simulink model "Stop_Model"  (R2023a)
settings: Solver=VariableStepAuto  StartTime=0.0  StopTime=10.0  RelTol=1e-3
libraries: TimeSharedLib x2, NSA_DEVS_SINKS_ATOMIC x2, NSA_DEVS_SOURCES_ATOMIC x1, NSA_DEVS_LOGISTICS_ATOMIC x1
settings Model: Creator=david  LastModifiedBy=peter

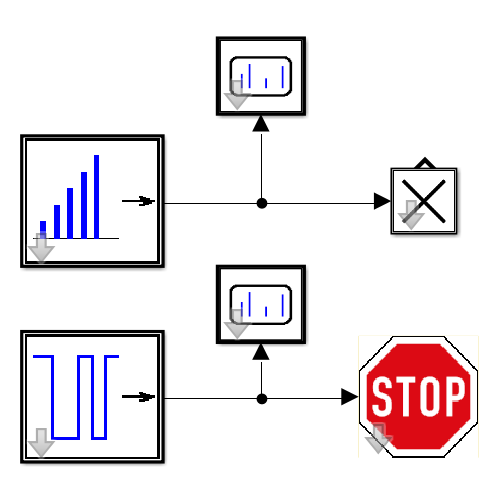
[thumbnail: Simulink's stored preview of the top-level diagram]
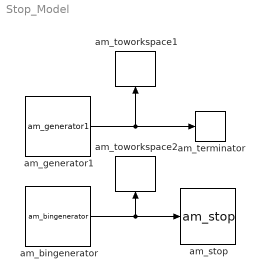
== system Stop_Model ==
  am_bingenerator : NSA_DEVS_SOURCES_ATOMIC/am_bingenerator  z0="\"0\""  tVec=[7.5]  tau=[0,1]  debug=0
      settings: SourceProductName=NSA_DEVS
  am_generator1 : TimeSharedLib/am_generator1  tG=1  n0=1  nG=10  tD=[0,2]  debug=0
  am_stop : TimeSharedLib/am_stop  tau=[0,1]  debug=0
  am_terminator : NSA_DEVS_LOGISTICS_ATOMIC/am_terminator  tau=[0,1]  debug=0
      settings: SourceProductName=NSA_DEVS
  am_toworkspace1 : NSA_DEVS_SINKS_ATOMIC/am_toworkspace  varname="\"dataOut\""  t0=0  format="\"vector\""  tau=[0,3]  debug=0
      settings: SourceProductName=NSA_DEVS
  am_toworkspace2 : NSA_DEVS_SINKS_ATOMIC/am_toworkspace  varname="\"binOut\""  t0=0  format="\"vector\""  tau=[0,3]  debug=0
      settings: SourceProductName=NSA_DEVS
  wires:
  am_generator1/1 -> am_terminator/1, am_toworkspace1/1
  am_bingenerator/1 -> am_toworkspace2/1, am_stop/1
